simulink model "Day14"  (R2024b)
settings: Solver=VariableStepAuto  StartTime=0.0  StopTime=10.0  RelTol=1e-3
settings Model: Creator=jun_mac  LastModifiedBy=jun_mac

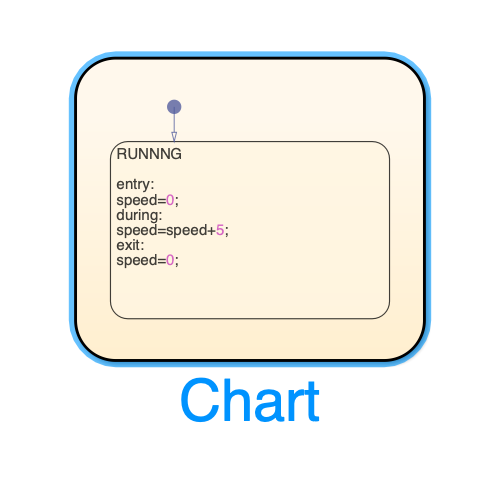
[thumbnail: Simulink's stored preview of the top-level diagram]
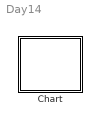
== system Day14 ==
  Chart : Stateflow chart  TreatAsAtomicUnit=on

== stateflow chart Day14/Chart ==
  state RUNNNG
    entry:
    speed=0;
    during:
    speed=speed+5;
    exit:
    speed=0;
  (default) -> RUNNNG
